simulink model "SPMe_CC_2023a"  (R2023a)
settings: Solver=VariableStepAuto  StartTime=0.0  StopTime=t_end  MaxStep=1  RelTol=1e-6
values from neighbouring files (symbols this model uses):
  dt = 0.05    [run_SPMe_sweep.m]
  I = 4.6*C_rates(c)    [run_SPMe_sweep.m]
  ocv_init = 4.2    [run_SPMe_sweep.m]
  V_min = 0    [run_SPMe_sweep.m]
undefined symbols (not defined in the file or in its folder): powergui, spspowerguiLib
libraries: spsControlledCurrentSourceLib x1, spsControlledVoltageSourceLib x1, spsCurrentMeasurementLib x1, spsParallelRLCBranchLib x1
settings Model: Creator=tom  LastModifiedBy=Vivian
settings SolverCC: AlgebraicLoopSolver=TrustRegion
settings DebuggingCC: UnconnectedInputMsg=warning  UnconnectedOutputMsg=warning  UnconnectedLineMsg=warning
settings ModelReferenceCC: EnableRefExpFcnMdlSchedulingChecks=on
settings RTWCC: DLArmComputeVersion=19.05

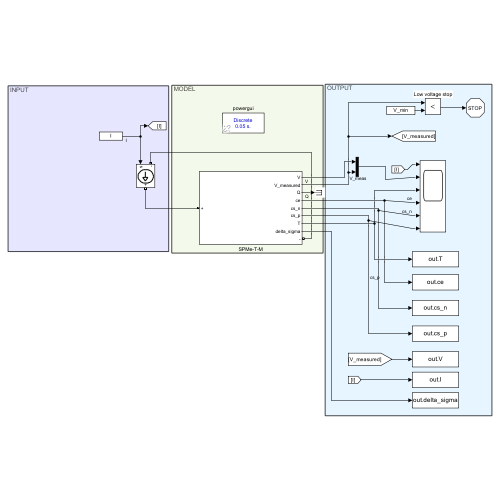
[thumbnail: Simulink's stored preview of the top-level diagram]
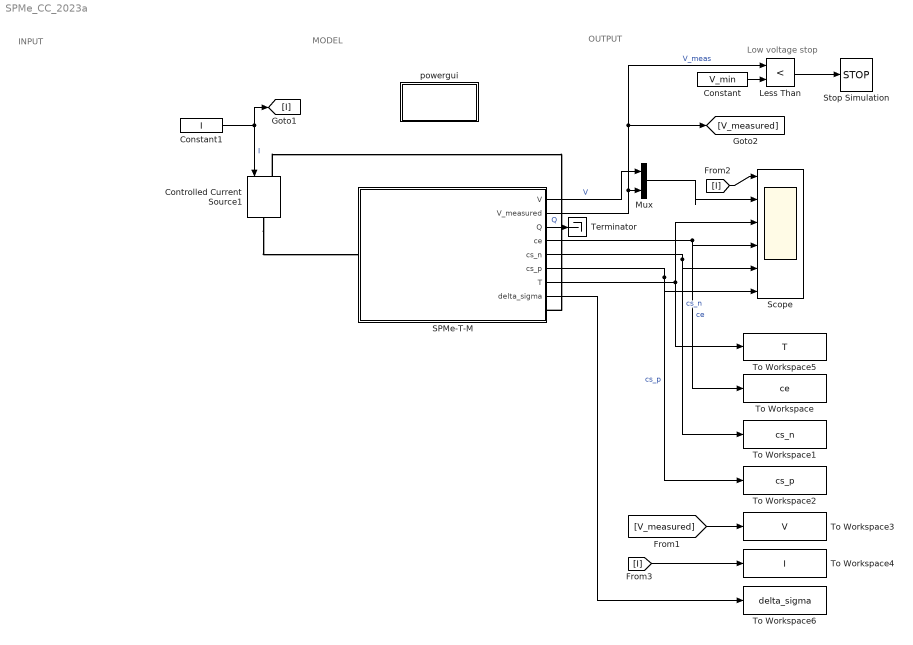
== system SPMe_CC_2023a ==
  note: OUTPUT
  note: MODEL
  note: INPUT
  note: Low voltage stop
  Constant : Constant  Value=V_min
  Constant1 : Constant  Value=I
  Controlled Current Source1 : spsControlledCurrentSourceLib/Controlled Current Source  Initialize=on  Source_Type=DC  Amplitude=0  Phase=0  Frequency=0  Measurements=None
  Less Than : RelationalOperator  Operator=<  OutDataTypeStr=boolean  RndMeth=Simplest  InputSameDT=off
  Mux : Mux  Inputs=2
  SPMe-T-M : Subsystem
  Scope : Scope  NumInputPorts=6
  Stop Simulation : Stop
  Terminator : Terminator
  To Workspace : ToWorkspace  VariableName=ce  SaveFormat=Timeseries  SampleTime=-1
  To Workspace1 : ToWorkspace  VariableName=cs_n  SaveFormat=Timeseries  SampleTime=-1
  To Workspace2 : ToWorkspace  VariableName=cs_p  SaveFormat=Timeseries  SampleTime=-1
  To Workspace3 : ToWorkspace  VariableName=V  SaveFormat=Timeseries  SampleTime=-1
  To Workspace4 : ToWorkspace  VariableName=I  SaveFormat=Timeseries  SampleTime=-1
  To Workspace5 : ToWorkspace  VariableName=T  SaveFormat=Timeseries  SampleTime=-1
  To Workspace6 : ToWorkspace  VariableName=delta_sigma  SaveFormat=Timeseries  SampleTime=-1
  powergui : Subsystem  Priority=1  AncestorBlock=spspowerguiLib/powergui  DialogController=POWERSYS.PowerSysDialog  InitFcn=powergui( 'InitFcn_Callback' , gcb , 0 , [ ] );  mask(PSB option menu block){SimulationMode=Discrete, SampleTime=dt, frequency=60, Iterations=50, frequencyindice=0, Pbase=100e6, ErrMax=1e-4, UnitsV=kV, UnitsW=MW, buscounter=0, FunctionMessages=off, echomessages=off, EnableUseOfTLC=off, CurrentSourceSwitches=off, DisableSnubberDevices=off, DisableRonSwitches=off, DisableVfSwitches=off, DisplayEquations=off, AutomaticDiscreteSolvers=off, SolverType=Tustin/Backward Euler (TBE), Interpol=off, ExternalGateDelay=off, methode=off, Ts=100, x0status=blocks, SPID=on, SwTol=0, HookPort=off, NonlinearTolerance=1e-4, nMaxIteration=100, ContinueOnMaxIteration=off, RestoreLinks=warning, ResistiveCurrentMeasurement=off, Frange=[0:2:500], Ylog=off, Xlog=on, ShowGrid=off, save=off, variable=ZData, structure=0, ZoomFFT=off, StartTime=0.0, cycles=1, DisplayStyle=1, fundamental=60, FreqAxis=off, MaxFrequency=1000, frequencyindicesteady=1, RmsSteady=1, display=off}
      mask prompts: SimulationMode "Simulation type:"; SampleTime "Sample time (s):"; frequency "Frequency (Hz):"; Iterations "Max iterations"; frequencyindice "Frequency (Hz)"; Pbase "Base power (VA)"; ErrMax "PQ tolerance (pu)"; UnitsV "Voltage units"; UnitsW "Power units"; buscounter "Load flow bus counter"; FunctionMessages "Disable Specialized Power Systems warnings"; echomessages "Display Specialized Power Systems compilation messages"; EnableUseOfTLC "Use TLC file when in Accelerator Simulation Mode and for code generation"; CurrentSourceSwitches "Disable ideal switching"; DisableSnubberDevices "Disable snubbers in switching devices"; DisableRonSwitches "Disable Ron resistances in switching devices"; DisableVfSwitches "Disable forward voltages in switching devices"; DisplayEquations "Display circuit differential equations"; AutomaticDiscreteSolvers "Automatically handle Discrete solver and Advanced tab solver settings of blocks"; SolverType "Discrete solver"; Interpol "Interpolate switching events"; ExternalGateDelay "Use time-stamped gate signals"; methode "Store switching topologies"; Ts "Buffer size (MBytes):"; x0status "Start simulation with initial electrical states from:"; SPID "Use ideal switching devices"; SwTol "Switch tolerance"; HookPort "Allow multiple powergui blocks"; NonlinearTolerance "Solver tolerance"; nMaxIteration "Maximum number of iterations"; ContinueOnMaxIteration "Continue Simulation if maximum number of iterations is reached"; RestoreLinks "Restore disabled links of Simscape Power Systems ST blocks:"; ResistiveCurrentMeasurement "Use non ideal current measurement blocks (1e-4Ohm internal resistance)"; Frange "Frequency Range"; Ylog "Log impedance"; Xlog "log Frequency"; ShowGrid "grid"; save "Save Data To Workspace"; variable "Variable Name"; structure "Structure Name (PSBFFTSCOPE)"; ZoomFFT "ZoomFFT (PSBFFTSCOPE)"; StartTime "Start Time (PSBFFTSCOPE)"; cycles "Cycles (PSBFFTSCOPE)"; DisplayStyle "Display style (PSBFFTSCOPE)"; fundamental "Fundamental (PSBFFTSCOPE)"; FreqAxis "Frequency Axis (PSBFFTSCOPE)"; MaxFrequency "Max Frequency (PSBFFTSCOPE)"; frequencyindicesteady "Frequency indice (STEADYSTATE)"; RmsSteady "RMS display (STEADYSTATE)"; display "Display Results"
      mask help: Set simulation type, simulation parameters, and preferences.
      mask init:
      | dispMessage = '';
      | dispMessage = powergui('MaskInitialization',gcb,SimulationMode,SampleTime);
      settings: PreSaveFcn=powergui( 'PreSaveFcn_Callback' , gcb , [ ] , [ ] );  OpenFcn=sps_rtmsupport('OpenFcn',gcbh)
      mask Help: helpview(psbhelp)
      mask TypeOptions SimulationMode: Continuous | Discrete | Phasor | Discrete phasor
      mask Callback SimulationMode: powergui('SimulationType',[],[],gcb);
      mask TypeOptions UnitsV: V | kV
      mask TypeOptions UnitsW: W | kW | MW
      mask Callback CurrentSourceSwitches: powergui('SimulationType',[],[],gcb);
      mask Callback AutomaticDiscreteSolvers: powergui('SimulationType',[],[],gcb);
      mask TypeOptions SolverType: Tustin/Backward Euler (TBE) | Tustin | Backward Euler
      mask Callback SolverType: powergui('SimulationType',[],[],gcb);
      mask Callback Interpol: powergui('SimulationType',[],[],gcb);
      mask Callback ExternalGateDelay: powergui('SimulationType',[],[],gcb);
      mask Callback methode: powergui('SimulationType',[],[],gcb);
      mask TypeOptions x0status: blocks | steady | zero
      mask TypeOptions RestoreLinks: yes | warning | no
      mask Callback display: sps_rtmsupport('parametereditingmodes',gcbh) % Will be executed last in parameter callbacks to ensure mask enable consistency
      mask DialogControl SolverTab Prompt: Solver
      mask DialogControl AutoSolverNote Prompt: The Simulation type parameter is governed by Simulink. To access the Powergui solver settings, unselect auto (Automatic solver selection) solver in the Simulink solver options.
      mask DialogControl Apps Prompt: Apps
      mask DialogControl StateAnalyzer Prompt: Measurements and States Analyzer
      mask DialogControl StateAnalyzer Callback: powerStates(bdroot(gcb))
      mask DialogControl LineParameterCalculator Prompt: Line Parameter Calculator
      mask DialogControl LineParameterCalculator Callback:
      | close_system(gcb)
      | powerLineParameters
      mask DialogControl CableParameterCalculator Prompt: Cable Parameter Calculator
      mask DialogControl CableParameterCalculator Callback:
      | close_system(gcb)
      | powerCableParameters
      mask DialogControl LineDecoupler Prompt: Line Decoupler
      mask DialogControl LineDecoupler Tooltip: Click to replace selected Distributed Parameters Line blocks with Decoupling Line blocks
      mask DialogControl LineDecoupler Callback:
      | close_system(gcb);
      | DecouplingLineReplace(gcs)
      mask DialogControl LoadFlowAnalyzer Prompt: Load Flow Analyzer
      mask DialogControl LoadFlowAnalyzer Callback:
      | close_system(gcb)
      | powerLoadFlow
      mask DialogControl LoadFlowParameters Prompt: Load Flow Parameters
      mask DialogControl ImpedanceCalculator Prompt: Impedance Calculator
      mask DialogControl ImpedanceCalculator Callback:
      | close_system(gcb);
      | powerImpedance(bdroot(gcs));
      mask DialogControl FFTAnalyzer Prompt: FFT Analyzer
      mask DialogControl FFTAnalyzer Callback:
      | close_system(gcb)
      | power_fftscope(bdroot(gcb),gcb)
      mask DialogControl LinearSystemAnalyzer Prompt: Linear System Analyzer
      mask DialogControl LinearSystemAnalyzer Callback:
      | close_system(gcb)
      | power_ltiview(bdroot(gcb))
      mask DialogControl HysteresisDesigner Prompt: Hysteresis Designer
      mask DialogControl HysteresisDesigner Callback:
      | close_system(gcb)
      | powerHysteresis('hysteresis.mat')
      mask DialogControl BlockCustomizer Prompt: Block Customizer
      mask DialogControl BlockCustomizer Callback:
      | close_system(gcb);
      | power_customize;
      mask DialogControl ReportGenerator Prompt: Report Generator
      mask DialogControl ReportGenerator Callback:
      | close_system(gcb)
      | power_report(bdroot(gcb))
      mask DialogControl obsolete Prompt: ...
      mask DialogControl MachineInitialization Prompt: Machine Initialization
      mask DialogControl MachineInitialization Callback:
      | close_system(gcb)
      | powericon('machineInitTool',bdroot(gcb),gcb)
      mask DialogControl Preferences Prompt: Preferences
      mask DialogControl Solver Prompt: Solver
      mask DialogControl SolverDetails Prompt: Solver details for nonlinear elements
      mask Display: color('blue'),disp(dispMessage)
  wires:
  SPMe-T-M/5(cs_n) -> To Workspace1/1, Scope/5  "cs_n"
  SPMe-T-M/6(cs_p) -> To Workspace2/1, Scope/6  "cs_p"
  Less Than/1 -> Stop Simulation/1
  Constant/1 -> Less Than/2
  SPMe-T-M/4(ce) -> To Workspace/1, Scope/4  "ce"
  SPMe-T-M/1(V) -> Mux/1  "V"
  SPMe-T-M/2(V_measured) -> Less Than/1, [V_measured], Mux/2  "V_meas"
  Constant1/1 -> Controlled Current Source1/1, [I]  "I"
  Mux/1 -> Scope/2
  [V_measured] -> To Workspace3/1
  [I] -> Scope/1
  [I] -> To Workspace4/1
  SPMe-T-M/8(delta_sigma) -> To Workspace6/1
  SPMe-T-M/3(Q) -> Terminator/1  "Q"
  SPMe-T-M/7(T) -> To Workspace5/1, Scope/3
  connections:
  Controlled Current Source1/RConn1 -- SPMe-T-M/LConn1
  Controlled Current Source1/LConn1 -- SPMe-T-M/RConn1

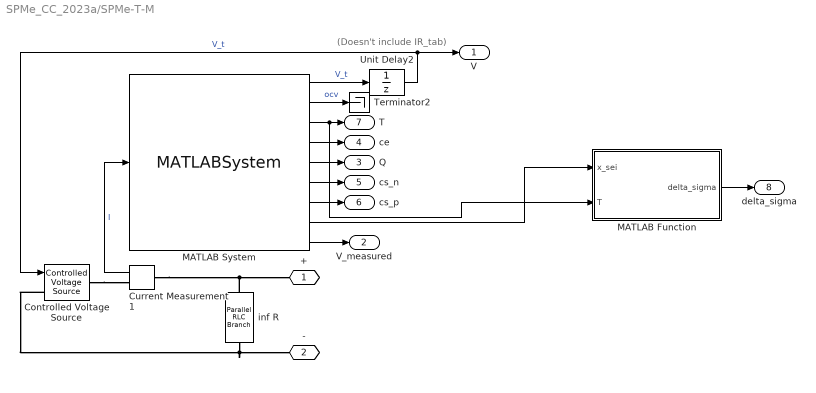
== system SPMe_CC_2023a/SPMe-T-M ==
  note: (Doesn't include IR_tab)
  Controlled Voltage Source : spsControlledVoltageSourceLib/Controlled Voltage Source  Initialize=on  Source_Type=AC  Amplitude=0  Phase=0  Frequency=0  Measurements=None
  Current Measurement1 : spsCurrentMeasurementLib/Current Measurement  PhasorSimulation=off  OutputType=Complex  PSBequivalent=0
  MATLAB Function : MATLAB Function  TreatAsAtomicUnit=on
  MATLAB System : MATLABSystem  System=pybamm_bat  SimulateUsing=Interpreted execution
      mask Type: pybamm_bat
      mask Display:
      | disp('pybamm_bat');
      | port_label('input',1,'current');
      | port_label('output',1,'V_t');
      | port_label('output',2,'ocv');
      | port_label('output',3,'T');
      | port_label('output',4,'ce');
      | port_label('output',5,'heating');
      | port_label('output',6,'neg_conc');
      | port_label('output',7,'pos_conc');
      | port_label('output',8,'x_sei');
      | port_label('output',9,'V_meas');
  Terminator2 : Terminator
  Unit Delay2 : UnitDelay  InitialCondition=ocv_init  SampleTime=-1  HasFrameUpgradeWarning=on
  inf R : spsParallelRLCBranchLib/Parallel RLC Branch  LConnTagsString=a  RConnTagsString=__new0  BranchType=R  Resistance=1e8  Inductance=1e-3  SetiL0=off  InitialCurrent=0  Capacitance=1e-6  Setx0=off  InitialVoltage=0  Measurements=None
  + : PMIOPort  Tag=PMCPort  Side=Left
  - : PMIOPort  Tag=PMCPort  Port=2  Side=Right
  V : Outport
  V_measured : Outport  Port=2
  Q : Outport  Port=3  VectorParamsAs1DForOutWhenUnconnected=off
  ce : Outport  Port=4
  cs_n : Outport  Port=5  VectorParamsAs1DForOutWhenUnconnected=off
  cs_p : Outport  Port=6  VectorParamsAs1DForOutWhenUnconnected=off
  T : Outport  Port=7
  delta_sigma : Outport  Port=8
  wires:
  Current Measurement1/1 -> MATLAB System/1  "I"
  MATLAB System/4 -> ce/1
  MATLAB System/5 -> Q/1
  MATLAB System/6 -> cs_n/1
  MATLAB System/7 -> cs_p/1
  MATLAB System/1 -> Unit Delay2/1  "V_t"
  Unit Delay2/1 -> V/1, Controlled Voltage Source/1  "V_t"
  MATLAB System/8 -> MATLAB Function/1(x_sei)
  MATLAB System/9 -> V_measured/1
  MATLAB System/3 -> MATLAB Function/2(T), T/1
  MATLAB System/2 -> Terminator2/1  "ocv"
  MATLAB Function/1(delta_sigma) -> delta_sigma/1
  connections:
  inf R/LConn1 -- +/RConn1 -- Current Measurement1/LConn1
  inf R/RConn1 -- Controlled Voltage Source/LConn1 -- -/RConn1
  Controlled Voltage Source/RConn1 -- Current Measurement1/RConn1

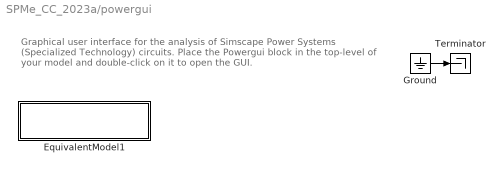
== system SPMe_CC_2023a/powergui ==
  note: Graphical user interface for the analysis of
      | Simscape Power Systems (Specialized Technology) circuits.
      | Place the Powergui block in the top-level of your model and double-click
      | on it to open the GUI.
  EquivalentModel1 : Subsystem
      mask init:
      | S  = GetDataForEquivalentModel('Discrete',gcbh);
      mask Display:
      | color('red')
      | disp('EQUIVALENT CIRCUIT\nDiscrete')
  Ground : Ground
  Terminator : Terminator
  wires:
  Ground/1 -> Terminator/1

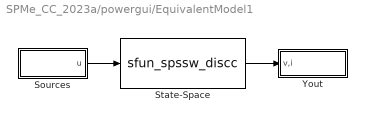
== system SPMe_CC_2023a/powergui/EquivalentModel1 ==
  Sources : Subsystem
  State-Space : S-Function  FunctionName=sfun_spssw_discc  Parameters=S.Ts,S.A, S.B, S.C, S.D, S.x0,S.EnableUseOfTLC  SFunctionDeploymentMode=off  EnableBusSupport=off
  Yout : Subsystem
  wires:
  State-Space/1 -> Yout/1(v,i)
  Sources/1(u) -> State-Space/1

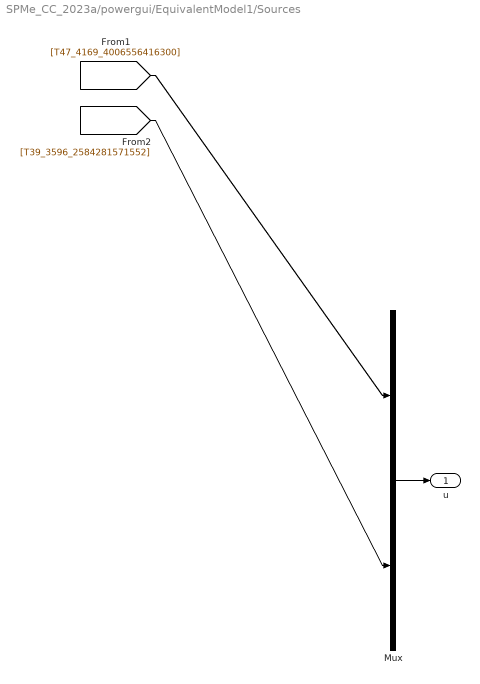
== system SPMe_CC_2023a/powergui/EquivalentModel1/Sources ==
  Mux : Mux  Inputs=[1 1]
  u : Outport  VectorParamsAs1DForOutWhenUnconnected=off
  wires:
  Mux/1 -> u/1
  [T47_4169_4006556416300] -> Mux/1
  [T39_3596_2584281571552] -> Mux/2

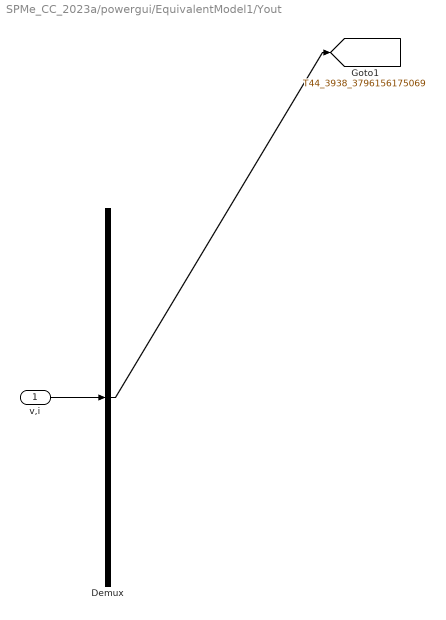
== system SPMe_CC_2023a/powergui/EquivalentModel1/Yout ==
  v,i : Inport
  Demux : Demux  Outputs=1
  tag scope: T44_3938_3796156175069=global
  wires:
  v,i/1 -> Demux/1
  Demux/1 -> [T44_3938_3796156175069]

== matlab function SPMe_CC_2023a/SPMe-T-M/MATLAB Function ==
  data: x_sei input; delta_sigma output; T input
function delta_sigma  = expansion(x_sei, T)
%XSEI2PTOTAL 
% Mechanical params
M_C6 = 72/1000; %kg/mol
% V_head_0 = 6.65e-6; %m3 (0.121*0.074*0.0055)*0.135
% L = 2.4/1000; %m
% E = 0.19e6; %Pa
% alpha_cell = 1.1e-6; %m/K
% P_atm = 101; %kPa
% P_crit = 158.7731; %kPa
R = 8.3145; %J.mol-1.K-1
A = 0.009; %m2 (0.121*0.074)
DMC = [6.4338; 1413; -44.25]; %Antoine coeffs [A B C] 
EC = [6.4897; 1836.57; -102.23];
y_dmc = 0.7;
y_ec = 1-y_dmc;         
m_an = 0.0191; 
x_sei_0 = 0.15;
% T_amb = 273.15+25; % K
% sigma_0 = 1.5120e+04;

% Internal cell pressure
V_head_0 = 6.65e-06; %m-3
L_p0 = 2.4e-3; %m for 2 poron
E_p = 0.19e6; %Pa Young's modulus for poron
% E_c = 1e12; %assume large by default
alpha = 1.1e-6; %m/K
P_atm = 101e3; %Pa
% P_crit = 158e3; %Pa
% P0 = 14e3; %Pa
R = 8.3145; %J.mol-1.K-1
% k_b = 1.380649e-23; %m2.kg.s-2.K-1;
T_amb = 273.15+25; % K
sigma_0 = 1.5120e+04;
% L_cs0 = 5.5e-3; %m initial cell solid thickness
% V_cell = 0.130*0.089*0.055; % [130mm×89mm×5.5mm] active material

% P_elyte
Psat_EC = 10.^(EC(1)-EC(2)./(EC(3)+T));
Psat_DMC = 10.^(DMC(1)-DMC(2)./(DMC(3)+T)); 
P_elyte = (y_dmc*Psat_DMC + y_ec*Psat_EC)*1e3; 

% P_CO2
n_CO2 = 0.5*m_an/M_C6*(x_sei_0-x_sei);

% Solve for gas volume and pressure
delta_sigma_calc = P_elyte - sigma_0 - P_atm;
a = 1;
b = -(V_head_0 + A.*(L_p0/E_p*(delta_sigma_calc) - alpha.*(T-T_amb)));
c = -A*L_p0/E_p.*n_CO2.*R.*(T);
V_g0 = (-b+sqrt(max(b.^2-4.*a.*c,0)))/(2*a);
V_g = max(V_g0, V_head_0); % min V_g = V_head_0

P_CO2 = n_CO2.*R.*T./V_g;
P_gas = P_elyte + P_CO2;

delta_sigma = max(P_gas-P_atm-sigma_0, E_p./L_p0.*alpha.*(T-T_amb));
end
